simulink model "discrete_model_nonlinear"  (R2023b)
settings: Solver=VariableStepAuto  StartTime=0.0  StopTime=t_fin  RelTol=1e-3
values from neighbouring files (symbols this model uses):
  a0 = 0.00376903    [model_setup.m]
  a1 = 0.0731193    [model_setup.m]
  a2 = 0.469961    [model_setup.m]
  alpha1 = 0.42    [model_setup.m]
  alpha2 = 0.19    [model_setup.m]
  alpha3 = 1.5    [model_setup.m]
  alpha4 = 0.95    [model_setup.m]
  b0 = 0.0050882    [model_setup.m]
  T = t_probing(j)    [ex8.m]    (also in model_setup.m = 0.1)
  u_max = u_maxs(i)    [ex6.m]    (also in ex8.m = 0.5; model_setup.m = 1)
  u_min = 0    [ex6.m]    (also in ex8.m; model_setup.m)
  u_step_time = 10    [model_setup.m]
settings Model: Creator=vistek528  LastModifiedBy=vistek528
settings DataIOCC: ReturnWorkspaceOutputs=off

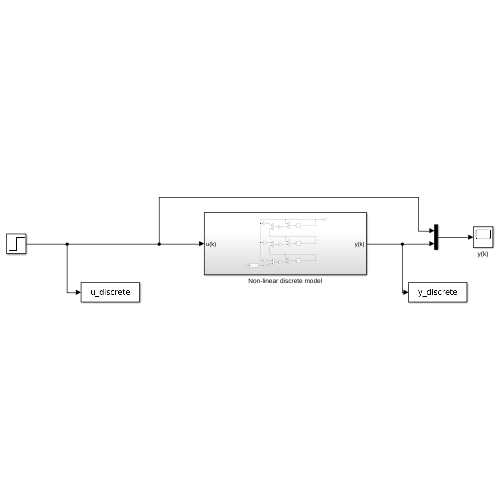
[thumbnail: Simulink's stored preview of the top-level diagram]
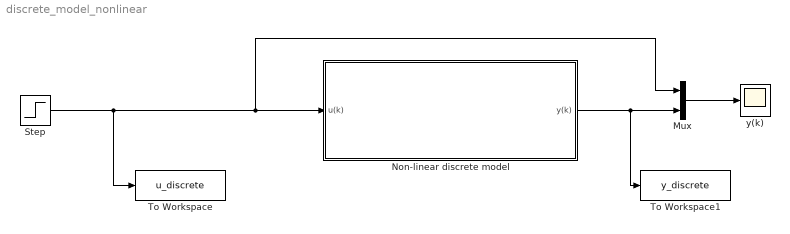
== system discrete_model_nonlinear ==
  Mux : Mux  Inputs=2
  Non-linear discrete model : Subsystem
  Step : Step  Time=u_step_time  Before=u_min  After=u_max  SampleTime=0
  To Workspace : ToWorkspace  VariableName=u_discrete  SaveFormat=Timeseries  SampleTime=-1
  To Workspace1 : ToWorkspace  VariableName=y_discrete  SaveFormat=Timeseries  SampleTime=-1
  y(k) : Scope
  wires:
  Step/1 -> To Workspace/1, Mux/1, Non-linear discrete model/1(u(k))
  Non-linear discrete model/1(y(k)) -> Mux/2, To Workspace1/1
  Mux/1 -> y(k)/1

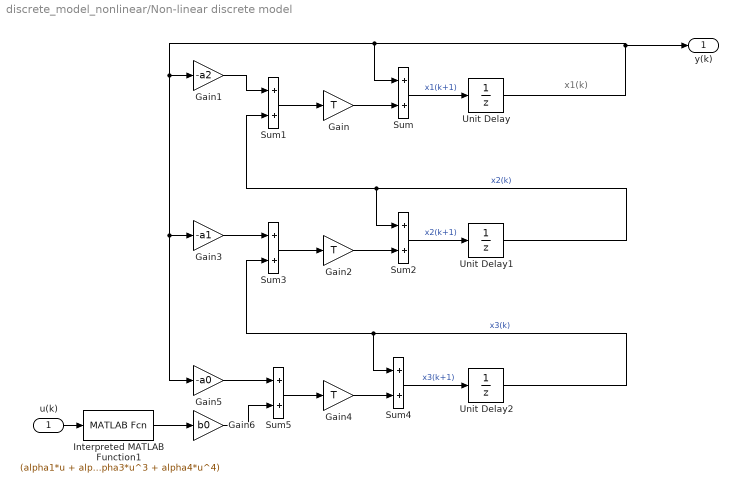
== system discrete_model_nonlinear/Non-linear discrete model ==
  note: x1(k)
  u(k) : Inport
  Gain : Gain  Gain=T
  Gain1 : Gain  Gain=-a2
  Gain2 : Gain  Gain=T
  Gain3 : Gain  Gain=-a1
  Gain4 : Gain  Gain=T
  Gain5 : Gain  Gain=-a0
  Gain6 : Gain  Gain=b0
  Interpreted MATLAB Function1 : MATLABFcn  MATLABFcn=(alpha1*u + alpha2*u^2 + alpha3*u^3 + alpha4*u^4)
  Sum{,1..5} (6 alike) : Sum
  Unit Delay : UnitDelay  SampleTime=T  HasFrameUpgradeWarning=on
  Unit Delay1 : UnitDelay  SampleTime=T  HasFrameUpgradeWarning=on
  Unit Delay2 : UnitDelay  SampleTime=T  HasFrameUpgradeWarning=on
  y(k) : Outport
  wires:
  u(k)/1 -> Interpreted MATLAB Function1/1
  Gain1/1 -> Sum1/1
  Gain5/1 -> Sum5/1
  Sum4/1 -> Unit Delay2/1  "x3(k+1)"
  Gain6/1 -> Sum5/2
  Gain/1 -> Sum/2
  Gain4/1 -> Sum4/2
  Interpreted MATLAB Function1/1 -> Gain6/1
  Gain3/1 -> Sum3/1
  Sum5/1 -> Gain4/1
  Gain2/1 -> Sum2/2
  Sum2/1 -> Unit Delay1/1  "x2(k+1)"
  Sum/1 -> Unit Delay/1  "x1(k+1)"
  Unit Delay1/1 -> Sum2/1, Sum1/2  "x2(k)"
  Sum3/1 -> Gain2/1
  Sum1/1 -> Gain/1
  Unit Delay2/1 -> Sum3/2, Sum4/1  "x3(k)"
  Unit Delay/1 -> Gain5/1, Gain3/1, Gain1/1, Sum/1, y(k)/1
